simulink model "LQR_State_Space"  (R2020a)
settings: Solver=VariableStepAuto  StartTime=0.0  StopTime=50  RelTol=1e-3
values from neighbouring files (symbols this model uses):
  A = [ 0 0 0 1 0 0;0 0 0 0 1 0;0 0 0 0 0 1 ... (first row only)    [LQR_controller_custom.m]    (also in plotter_custom.m)
  B = [ 0 0 0;0 0 0;0 0 0; 0.102 0 0; 0 0.103 0; 0 0 0.103]    [LQR_controller_custom.m]    (also in plotter_custom.m)
  C = [ 0 0 0 0 0 0;0 0 0 0 0 0;0 0 0 0 0 0 ... (first row only)    [LQR_controller_custom.m]    (also in plotter_custom.m)
  D = [ 0 0 0;0 0 0;0 0 0; 0 0 0;0 0 0;0 0 0]    [LQR_controller_custom.m]    (also in plotter_custom.m)
undefined symbols (not defined in the file or in its folder): K
settings Model: Creator=siddh  LastModifiedBy=siddh
settings DataIOCC: ReturnWorkspaceOutputs=off

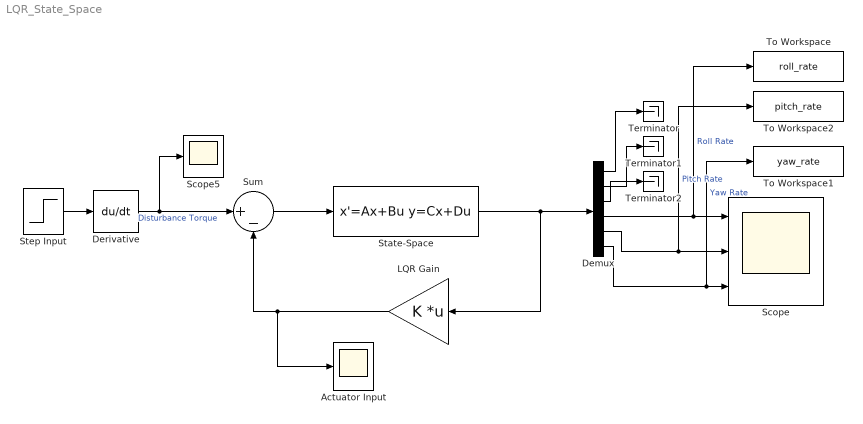
== system LQR_State_Space ==
  Actuator Input : Scope
  Demux : Demux  Outputs=6
  Derivative : Derivative
  LQR Gain : Gain  Gain=K  Multiplication=Matrix(K*u)
  Scope : Scope  NumInputPorts=3
  Scope5 : Scope
  State-Space : StateSpace  A=A  B=B  C=C  D=D  InitialCondition=[3 1 1 0 0 0]'
  Step Input : Step  SampleTime=0
  Sum : Sum  Inputs=|+-
  Terminator : Terminator
  Terminator1 : Terminator
  Terminator2 : Terminator
  To Workspace : ToWorkspace  VariableName=roll_rate  SaveFormat=Timeseries  SampleTime=-1
  To Workspace1 : ToWorkspace  VariableName=yaw_rate  SaveFormat=Timeseries  SampleTime=-1
  To Workspace2 : ToWorkspace  VariableName=pitch_rate  SaveFormat=Timeseries  SampleTime=-1
  wires:
  State-Space/1 -> Demux/1, LQR Gain/1
  LQR Gain/1 -> Sum/2, Actuator Input/1
  Sum/1 -> State-Space/1
  Demux/4 -> To Workspace/1, Scope/1  "Roll Rate"
  Step Input/1 -> Derivative/1
  Derivative/1 -> Scope5/1, Sum/1  "Disturbance Torque"
  Demux/5 -> To Workspace2/1, Scope/2  "Pitch Rate"
  Demux/6 -> To Workspace1/1, Scope/3  "Yaw Rate"
  Demux/3 -> Terminator2/1
  Demux/2 -> Terminator1/1
  Demux/1 -> Terminator/1
